simulink model "MATE_IEEE13Node"  (R2024b)
settings: Solver=FixedStepDiscrete  StartTime=0.0  StopTime=1  FixedStep=Ts  MaxStep=0.04  RelTol=1e-3
PostLoadFcn:
  | Ts=25e-6;
  | ieee_13NodesTestFeeder_init;
InitFcn:
  | Ts=25e-6;
  | ieee_13NodesTestFeeder_init;
undefined symbols (not defined in the file): C_603, C_604, C_605, C_607, ft2km, ieee_13NodesTestFeeder_init, L_603, L_604, L_605, L_607, R_603, R_604, R_605, R_607
libraries: simetranss x39, ee_lib x13, fl_lib x3, nesl_utility x3
Description:
  | Copyright 2008-2017 The MathWorks, Inc.
settings Model: ModifiedByFormat=Kyle Diller  Creator=Kyle Diller  LastModifiedBy=Kyle Diller
settings SolverCC: AlgebraicLoopSolver=TrustRegion
settings DataIOCC: ExternalInput=getinputstruct(op_IEEE_13_node_5)  InitialState=getstatestruct(op_IEEE_13_node_5)  LimitDataPoints=on  SaveFormat=Array  SignalLoggingSaveFormat=ModelDataLogs  ReturnWorkspaceOutputs=off
settings OptimizationCC: ExpressionDepthLimit=2147483647  LifeSpan=inf
settings DebuggingCC: AlgebraicLoopMsg=none  UnderspecifiedInitializationDetection=Classic  MergeDetectMultiDrivingBlocksExec=none  FcnCallInpInsideContextMsg=warning  AllowSymbolicDim=off  StateNameClashWarn=warning  SFUnexpectedBacktrackingDiag=warning  SFNoUnconditionalDefaultTransitionDiag=warning  SFExecutionAtInitializationDiag=none  ArithmeticOperatorsInVariantConditions=warning
settings HardwareCC: ProdBitPerPointer=32  ProdBitPerSizeT=32  ProdBitPerPtrDiffT=32  ProdLargestAtomicFloat=None  ProdIntDivRoundTo=Undefined  ProdEndianess=Unspecified  ProdWordSize=32  ProdHWDeviceType=32-bit Generic
settings ModelReferenceCC: EnableRefExpFcnMdlSchedulingChecks=on  PropagateSignalLabelsOutOfModel=off
settings SFSimCC: SimUseLocalCustomCode=off  CustomCodeUndefinedFunction=UseInterfaceOnly
settings RTWCC: RTWUseLocalCustomCode=off  GPUComputeCapability=3.5
settings CodeAppCC: StateflowObjectComments=on
settings GRTTargetCC: TargetLangStandard=C89/C90 (ANSI)  CombineOutputUpdateFcns=off  GRTInterface=on
settings ConfigComp: CovMetricSettings=dw  CovSaveCumulativeToWorkspaceVar=on  CovSaveSingleToWorkspaceVar=on  CovExternalEMLEnable=off  CovSFcnEnable=off
settings SimscapeCC: SimscapeNormalizeSystem=off

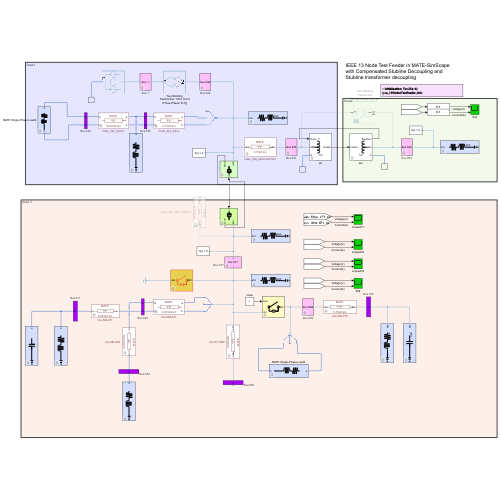
[thumbnail: Simulink's stored preview of the top-level diagram]
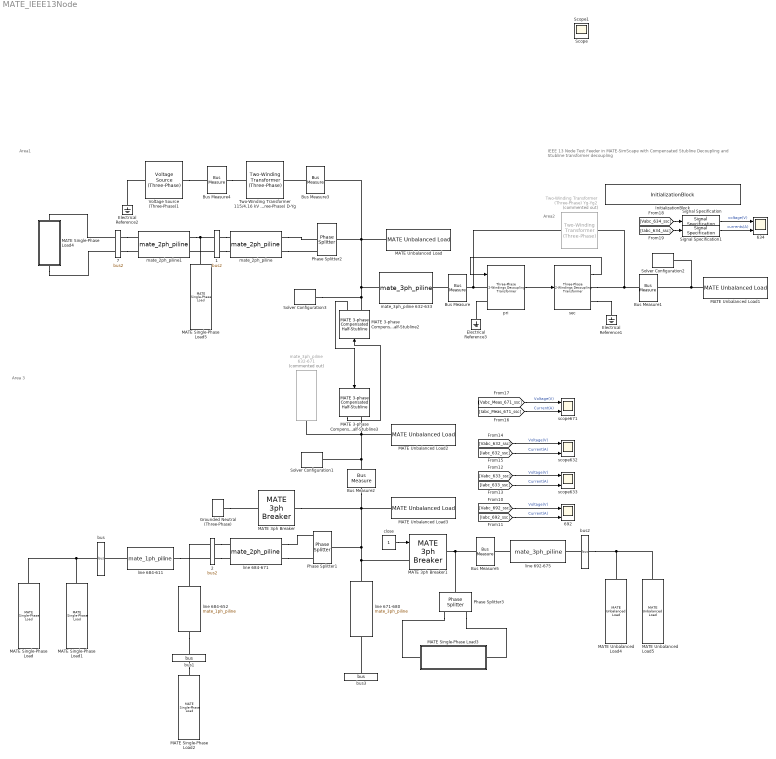
== system MATE_IEEE13Node ==
  note: IEEE 13 Node Test Feeder in MATE-SimScape
      | with Compensated Stubline Decoupling and
      | Stubline transformer decoupling
  note: Area1
  note: Area2
  note: Area 3
  1 : simetranss/Measure/bus2  bn=645
      settings: AttributesFormatString=Bus %<bn>
  2 : simetranss/Measure/bus2  bn=684
      settings: AttributesFormatString=Bus %<bn>
  634 : Scope  NumInputPorts=2
  692 : Scope  NumInputPorts=2
  7 : simetranss/Measure/bus2  bn=646
      settings: AttributesFormatString=Bus %<bn>
  Bus Measure : simetranss/Measure/Bus Measure  VoltageMeasurement=phase-to-phase  SetLabelV=on  LabelV=Vabc_633_ssc  Vpu=off  VpuLL=off  CurrentMeasurement=yes  SetLabelI=on  LabelI=Iabc_633_ssc  Ipu=off  Pbase=100e6  Vbase=500e3  bnumber=633  dis=off
      settings: AttributesFormatString=Bus %<bnumber>
  Bus Measure1 : simetranss/Measure/Bus Measure  VoltageMeasurement=phase-to-phase  SetLabelV=on  LabelV=Vabc_634_ssc  Vpu=off  VpuLL=off  CurrentMeasurement=yes  SetLabelI=on  LabelI=Iabc_634_ssc  Ipu=off  Pbase=100e6  Vbase=500e3  bnumber=634  dis=off
      settings: AttributesFormatString=Bus %<bnumber>
  Bus Measure2 : simetranss/Measure/Bus Measure  VoltageMeasurement=phase-to-ground  SetLabelV=on  LabelV=Vabc_Meas_671_ssc  Vpu=off  VpuLL=off  CurrentMeasurement=yes  SetLabelI=on  LabelI=Iabc_Meas_671_ssc  Ipu=off  Pbase=100e6  Vbase=500e3  bnumber=671  dis=off
      settings: AttributesFormatString=Bus %<bnumber>
  Bus Measure3 : simetranss/Measure/Bus Measure  VoltageMeasurement=phase-to-ground  SetLabelV=on  LabelV=Vabc_632_ssc  Vpu=off  VpuLL=off  CurrentMeasurement=yes  SetLabelI=on  LabelI=Iabc_632_ssc  Ipu=off  Pbase=100e6  Vbase=500e3  bnumber=632  dis=off
      settings: AttributesFormatString=Bus %<bnumber>
  Bus Measure4 : simetranss/Measure/Bus Measure  VoltageMeasurement=phase-to-ground  SetLabelV=on  LabelV=V1  Vpu=off  VpuLL=off  CurrentMeasurement=yes  SetLabelI=on  LabelI=I1  Ipu=off  Pbase=100e6  Vbase=500e3  bnumber=1  dis=off
      settings: AttributesFormatString=Bus %<bnumber>
  Bus Measure5 : simetranss/Measure/Bus Measure  VoltageMeasurement=phase-to-ground  SetLabelV=on  LabelV=Vabc_692_ssc  Vpu=off  VpuLL=off  CurrentMeasurement=yes  SetLabelI=on  LabelI=Iabc_692_ssc  Ipu=off  Pbase=100e6  Vbase=500e3  bnumber=692  dis=off
      settings: AttributesFormatString=Bus %<bnumber>
  Electrical Reference1 : fl_lib/Electrical/Electrical Elements/Electrical Reference
  Electrical Reference2 : fl_lib/Electrical/Electrical Elements/Electrical Reference
  Electrical Reference3 : fl_lib/Electrical/Electrical Elements/Electrical Reference
  Grounded Neutral (Three-Phase) : ee_lib/Connectors & References/Grounded Neutral (Three-Phase)
  InitializationBlock : simetranss/Usefulls/InitializationBlock  InitVar=Ts=25e-6;  InitFile=ieee_13NodesTestFeeder_init;  prel=off  posl=on  inif=on
  MATE 3-phase Compensated Half-Stubline2 : simetranss/Network decoupling/MATE 3-phase Compensated Half-Stubline  stype=3-phase coupled line (1 mode)  FF=60  RR=R_601  LL=L_601  CC=C_601  len=2000*ft2km  Ts=Ts  comp=on  stdel=off
  MATE 3-phase Compensated Half-Stubline3 : simetranss/Network decoupling/MATE 3-phase Compensated Half-Stubline  stype=3-phase coupled line (1 mode)  FF=60  RR=R_601  LL=L_601  CC=C_601  len=2000*ft2km  Ts=Ts  comp=off  stdel=off
  MATE 3ph Breaker : simetranss/Switches/MATE 3ph Breaker  InitialState=open  SwitchA=on  SwitchB=off  SwitchC=off  SwitchTimes=[0.2 0.25]  External=off  BreakerResistance=0.01  Roff=1e9  SnubberResistance=1e6  SnubberCapacitance=inf
  MATE 3ph Breaker1 : simetranss/Switches/MATE 3ph Breaker  InitialState=open  SwitchA=on  SwitchB=off  SwitchC=off  SwitchTimes=[0.2 0.25]  External=on  BreakerResistance=0.01  Roff=0  SnubberResistance=1e6  SnubberCapacitance=inf
  MATE Single-Phase Load : simetranss/Passive/MATE Single-Phase Load  Vabc=4160/sqrt(3)  Fn=60  typ=Capacitance  Pabc=[160 ]*1e3  QLabc=[ 90]*1e3  QCabc=100e3
  MATE Single-Phase Load1 : simetranss/Passive/MATE Single-Phase Load  Vabc=4160/sqrt(3)  Fn=60  typ=Series RL  Pabc=170e3  QLabc=80e3  QCabc=100e3
  MATE Single-Phase Load2 : simetranss/Passive/MATE Single-Phase Load  Vabc=4160/sqrt(3)  Fn=60  typ=Series RL  Pabc=128e3  QLabc=86e3  QCabc=100e3
  MATE Single-Phase Load3 : Subsystem  AncestorBlock=simetranss/Passive/MATE Single-Phase Load  mask(MATE 1-phase load){Vabc=1.71484*2401.78, Fn=60, typ=Series RL, Pabc=170e3, QLabc=151e3, QCabc=100e3}
      mask prompts: Vabc "Nominal voltage (Vrms)"; Fn "Nominal frequency fn (Hz):"; typ "Load type"; Pabc "Active powers (W)"; QLabc "Inductive reactive powers (positive var):"; QCabc "Capacitive reactive powers (positive var):"
      mask help: This block implements either a series RL load or a purely capacitive load.
      mask init:
      | block=gcb;
      | type=get_param(block,'typ');
      | 
      | if isequal (type,'Series RL')
      | j=sqrt(-1);
      | S=Pabc-j*QLabc;
      | Z=Vabc.*Vabc./S;
      | R=real(Z);
      | L=imag(Z)/2/pi/Fn;
      | 
      | s1 = 0;
      | s2 =-50;
      | s3 = 450;
      | s4 =50;
      | r1 = [0    30    30    38    53    68    83    98   113   120   120   150];
      | r2 =[0     0     0    25   -25    25   -25    25   -25     0     0     0];
      | c1 =[0];
      | c2 =[0 ];
      | c3 =[0];
      | c4 = [0];
      | c5=0;
      | c6=0;
      | l1 =[150   173   173   174   178   184   190   197   202   205   206   204   201 201   197   196   198   201   207   214   220   225   229   229   227   224   224   220   219   221   225   230   237   243   249   252   253   251   247  247   244   243   244   248   254   260   267   272   275   276   276   300 450];
      | l2 =[0     0     1    11    19    24    25    23    17     8    -2   -12   -18 -18    -9     1    11    19    24    25    23    17     8    -2   -12   -18 -18    -9     1    11    19    24    25    23    17     8    -2   -12   -18  -18    -9     1    11    19    24    25    23    17     8     0     0     0 0];
      | sca=0.5;
      | neutral=0;
      | ground=0;
      | else
      |     j=sqrt(-1);
      | S=QCabc;
      | Z=Vabc.*Vabc./S;
      | w=2*pi*Fn;
      | % Z=1/(wC)
      | C=1/w./Z;
      | 
      | 
      | s1 = 0;
      | s2 =-50;
      | s3 = 450;
      | s4 =50;
      | r1 = [0    ];
      | r2 =[0   ];
      | c1 =[450   390   390   393   395   393   390   390   393   395]-200;
      | c2 =[0     0     8    16    25    16     8    -8   -16   -25];
      | c3 =[360   360   360   250]-200;
      | c4 = [25   -25     0     0];
      | c5 =[ 455 200];
      | c6 = [0 0];
      | l1 =[0];
      | l2 =[0 ];
      | sca=0.5;
      | neutral=0;
      | 
      | ground=1;
      | 
      | 
      | 
      | end
      mask TypeOptions typ: Series RL | Capacitance
      mask Callback typ:
      | block = gcb;
      | type=get_param(block,'typ');
      | 
      | visib=get_param(block,'MaskVisibilities');
      | if isequal(type,'Series RL')
      |     visib{4}='on';;visib{5}='on';visib{6}='off';
      | else
      |     visib{4}='off';visib{5}='off';visib{6}='on';
      | end
      | set_param(block,'MaskVisibilities',visib);
      | 
      | 
      | if isequal(type,'Series RL')
      |     set_param([block '/RLseries'], 'Commented', 'off');
      |     set_param([block '/C'], 'Commented', 'on');
      | else
      |     set_param([block '/RLseries'], 'Commented', 'on');
      |     set_param([block '/C'], 'Commented', 'off');
      | end
      mask Display:
      | plot(s1-160,s2,s3+80,s4,r1,r2,l1,l2,c1,c2,c3,c4,c5,c6)
      | 
      | plot( ground*[s3,s3], ground*[-s2/4,s2/4])
      | plot( ground*[s3+30,s3+30], ground*[-s2/6,s2/6])
      | plot( ground*[s3+60,s3+60], ground*[-s2/10,s2/10])
      | 
      | plot( neutral*[s3,s3+80], neutral*[0,0])
  MATE Single-Phase Load4 : Subsystem  AncestorBlock=simetranss/Passive/MATE Single-Phase Load  mask(MATE 1-phase load){Vabc=4160, Fn=60, typ=Series RL, Pabc=170e3, QLabc=151e3, QCabc=100e3}
      mask prompts: Vabc "Nominal voltage (Vrms)"; Fn "Nominal frequency fn (Hz):"; typ "Load type"; Pabc "Active powers (W)"; QLabc "Inductive reactive powers (positive var):"; QCabc "Capacitive reactive powers (positive var):"
      mask help: This block implements either a series RL load or a purely capacitive load.
      mask init: same as MATE_IEEE13Node/MATE Single-Phase Load3
      mask TypeOptions typ: Series RL | Capacitance
      mask Callback typ:
      | block = gcb;
      | type=get_param(block,'typ');
      | 
      | visib=get_param(block,'MaskVisibilities');
      | if isequal(type,'Series RL')
      |     visib{4}='on';;visib{5}='on';visib{6}='off';
      | else
      |     visib{4}='off';visib{5}='off';visib{6}='on';
      | end
      | set_param(block,'MaskVisibilities',visib);
      | 
      | 
      | if isequal(type,'Series RL')
      |     set_param([block '/RLseries'], 'Commented', 'off');
      |     set_param([block '/C'], 'Commented', 'on');
      | else
      |     set_param([block '/RLseries'], 'Commented', 'on');
      |     set_param([block '/C'], 'Commented', 'off');
      | end
      mask Display:
      | plot(s1-160,s2,s3+80,s4,r1,r2,l1,l2,c1,c2,c3,c4,c5,c6)
      | 
      | plot( ground*[s3,s3], ground*[-s2/4,s2/4])
      | plot( ground*[s3+30,s3+30], ground*[-s2/6,s2/6])
      | plot( ground*[s3+60,s3+60], ground*[-s2/10,s2/10])
      | 
      | plot( neutral*[s3,s3+80], neutral*[0,0])
  MATE Single-Phase Load5 : simetranss/Passive/MATE Single-Phase Load  Vabc=1.03283*4160/sqrt(3)  Fn=60  typ=Series RL  Pabc=170e3  QLabc=125e3  QCabc=100e3
  MATE Unbalanced Load : simetranss/Passive/MATE Unbalanced Load  Vabc=[ 1.021 1.042 1.0174]*2401.78  Fn=60  typ=Series RL  Pabc="[17 66  117]*1e3/2"  QLabc="[10 38  68]*1e3/2"  QCabc="[190  60  212]*1e3"
  MATE Unbalanced Load1 : simetranss/Passive/MATE Unbalanced Load  Vabc=[ 0.993926 1.02168 0.995885]*277.128  Fn=60  typ=Series RL  Pabc=[160 120 120]*1e3  QLabc=[110 90 90]*1e3  QCabc="[190  60  212]*1e3"
  MATE Unbalanced Load2 : simetranss/Passive/MATE Unbalanced Load  Vabc=[ 0.987076 1.0519 0.978043]*2401.78  Fn=60  typ=Series RL  Pabc="[17 66  117]*1e3/2"  QLabc="[10 38  68]*1e3/2"  QCabc="[190  60  212]*1e3"
  MATE Unbalanced Load3 : simetranss/Passive/MATE Unbalanced Load  Vabc=[ 1.73773 1.77224 1.71484]*2401.78  Fn=60  typ=Series RL  Pabc=[385 385 385 ]*1e3  QLabc=[220 220 220]*1e3  QCabc="[190  60  212]*1e3"
  MATE Unbalanced Load4 : simetranss/Passive/MATE Unbalanced Load  Vabc=[ 0.98063 1.05431 0.975983]*2401.78  Fn=60  typ=Series RL  Pabc="[485  68  290]*1e3"  QLabc="[190  60  212]*1e3"  QCabc="[190  60  212]*1e3"
  MATE Unbalanced Load5 : simetranss/Passive/MATE Unbalanced Load  Vabc=[ 0.98063 1.05431 0.975983]*2401.78  Fn=60  typ=Capacitance  Pabc="[485  68  290]*1e3"  QLabc="[190  60  212]*1e3"  QCabc="[190  60  212]*1e3"
  Phase Splitter1 : ee_lib/Connectors & References/Phase Splitter
  Phase Splitter2 : ee_lib/Connectors & References/Phase Splitter
  Phase Splitter3 : ee_lib/Connectors & References/Phase Splitter
  Signal Specification : SignalSpecification  Dimensions=3
  Signal Specification1 : SignalSpecification  Dimensions=3
  Solver Configuration1 : nesl_utility/Solver Configuration  PhysicalDomain=network_engine_domain  SubClassName=solver  LeftPortType=input  RightPortType=generic  Tones=[]  Harmonics=[]  SimulateNoise=off  Profile=off  UseLocalSampling=off  EnableSwitchedLinearOptims=on  FrequencyDomain=off  UseCCode=off  RelTol=0.001  AbsTol=1e-06  MinStep=1e-09  ToWorkspace=off  RevertToSquareIcSolve=off  NumHomotopyIterations=100  PhasorMode=off  PhasorModeNumHarmonics=1  ConsistencySolver=NEWTON_FTOL  IndexReductionMethod=DerivativeReplacement  DoDC=off  ResidualTolerance=1e-09  ConsistencyTolSource=GLOBAL  ConsistencyAbsTol=0.001  ConsistencyRelTol=0.001  ConsistencyTolFactor=0.001  UseLocalSolver=on  LocalSolverChoice=NE_PARTITIONING_ADVANCER  ResolveIndetEquations=on  FunctionEvalNumThread=1  LocalSolverSampleTime=Ts  DoFixedCost=on  MaxNonlinIter=1  MaxModeIter=2  ComputeImpulses=off  ImpulseIterations=2  LinearAlgebra=auto  LinearAlgebraNumThread=0  EquationFormulation=NE_TIME_EF  DelaysMemoryBudget=1024  AutomaticFiltering=off  FilteringTimeConstant=0.001  PartitionStorageMethod=AS_NEEDED  PartitionMemoryBudget=1024  PartitionMethod=ROBUST  MultibodyUseLocalSolver=off  MultibodyLocalSolverChoice=ODE1  MultibodyLocalSolverSampleTime=0.001
  Solver Configuration2 : nesl_utility/Solver Configuration  PhysicalDomain=network_engine_domain  SubClassName=solver  LeftPortType=input  RightPortType=generic  Tones=[]  Harmonics=[]  SimulateNoise=off  Profile=off  UseLocalSampling=off  EnableSwitchedLinearOptims=on  FrequencyDomain=off  UseCCode=off  RelTol=0.001  AbsTol=1e-06  MinStep=1e-09  ToWorkspace=off  RevertToSquareIcSolve=off  NumHomotopyIterations=100  PhasorMode=off  PhasorModeNumHarmonics=1  ConsistencySolver=NEWTON_FTOL  IndexReductionMethod=DerivativeReplacement  DoDC=off  ResidualTolerance=1e-09  ConsistencyTolSource=GLOBAL  ConsistencyAbsTol=0.001  ConsistencyRelTol=0.001  ConsistencyTolFactor=0.001  UseLocalSolver=on  LocalSolverChoice=NE_PARTITIONING_ADVANCER  ResolveIndetEquations=on  FunctionEvalNumThread=1  LocalSolverSampleTime=Ts  DoFixedCost=on  MaxNonlinIter=1  MaxModeIter=2  ComputeImpulses=off  ImpulseIterations=2  LinearAlgebra=auto  LinearAlgebraNumThread=0  EquationFormulation=NE_TIME_EF  DelaysMemoryBudget=1024  AutomaticFiltering=off  FilteringTimeConstant=0.001  PartitionStorageMethod=AS_NEEDED  PartitionMemoryBudget=1024  PartitionMethod=ROBUST  MultibodyUseLocalSolver=off  MultibodyLocalSolverChoice=ODE1  MultibodyLocalSolverSampleTime=0.001
  Solver Configuration3 : nesl_utility/Solver Configuration  PhysicalDomain=network_engine_domain  SubClassName=solver  LeftPortType=input  RightPortType=generic  Tones=[]  Harmonics=[]  SimulateNoise=off  Profile=off  UseLocalSampling=off  EnableSwitchedLinearOptims=on  FrequencyDomain=off  UseCCode=off  RelTol=0.001  AbsTol=1e-06  MinStep=1e-09  ToWorkspace=off  RevertToSquareIcSolve=off  NumHomotopyIterations=100  PhasorMode=off  PhasorModeNumHarmonics=1  ConsistencySolver=NEWTON_FTOL  IndexReductionMethod=DerivativeReplacement  DoDC=off  ResidualTolerance=1e-09  ConsistencyTolSource=GLOBAL  ConsistencyAbsTol=0.001  ConsistencyRelTol=0.001  ConsistencyTolFactor=0.001  UseLocalSolver=on  LocalSolverChoice=NE_PARTITIONING_ADVANCER  ResolveIndetEquations=on  FunctionEvalNumThread=1  LocalSolverSampleTime=Ts  DoFixedCost=on  MaxNonlinIter=1  MaxModeIter=2  ComputeImpulses=off  ImpulseIterations=2  LinearAlgebra=auto  LinearAlgebraNumThread=0  EquationFormulation=NE_TIME_EF  DelaysMemoryBudget=1024  AutomaticFiltering=off  FilteringTimeConstant=0.001  PartitionStorageMethod=AS_NEEDED  PartitionMemoryBudget=1024  PartitionMethod=ROBUST  MultibodyUseLocalSolver=off  MultibodyLocalSolverChoice=ODE1  MultibodyLocalSolverSampleTime=0.001
  Two-Winding Transformer (Three-Phase) Yg-Yg2 : ee_lib/Passive/Transformers/Two-Winding Transformer (Three-Phase)  Commented=on  SRated=500e3 A*V  FRated=60 Hz  Winding1Connection=ee.enum.windingconnection.Yg  VRated1=4160 V  Winding2Connection=ee.enum.windingconnection.Yg  VRated2=480 V  CoreType=ee.enum.coretype.fivelimb  pu_Rw1=0.01  pu_Rw2=0.001  leakage_reactance_option=ee.enum.transformer_leakage.include  pu_Xl1=0.01  pu_Xl2=0.01  magnetizing_resistance_option=ee.enum.transformer_magnetizingResistance.exclude  pu_Rm=500  magnetizing_reactance_option=ee.enum.transformer_magnetizingReactance.exclude  saturation_option=ee.enum.transformer_saturation.exclude  pu_Xm=500  current_data=[0, .002, 1, 2]  magnetic_flux_data=[0, 1.2, 1.5, 1.51]  pu_X0=5000  i1_specify=off  i1_priority=None  i1=[0, 0, 0] A  i1_nominal_specify=off  i1_nominal_value=1  i1_nominal_unit=A  i2_specify=off  i2_priority=None  i2=[0, 0, 0] A  i2_nominal_specify=off  i2_nominal_value=1  i2_nominal_unit=A  phi_specify=off  phi_priority=None  phi=[0, 0, 0]  phi_nominal_specify=off  phi_nominal_value=1  phi_nominal_unit=1  power_dissipated_specify=off  power_dissipated_priority=None  power_dissipated=0 W  power_dissipated_nominal_specify=off  power_dissipated_nominal_value=1  power_dissipated_nominal_unit=W
      settings: InternalSimscapePortConfiguration="{\"Bottom\":[],\"Left\":[{\"id\":\"N1\",\"label\":\"~1\",\"type\":\"foundation.electrical.three_phase\"}],\"Right\":[{\"id\":\"N2\",\"label\":\"~2\",\"type\":\"foundation.electrical.three_phase\"}],\"Top\":[]}"
  Two-Winding Transformer 115/4.16 kV (Three-Phase) D-Yg : ee_lib/Passive/Transformers/Two-Winding Transformer (Three-Phase)  SRated=5000e3 A*V  FRated=60 Hz  Winding1Connection=ee.enum.windingconnection.delta1  VRated1=115e3 V  Winding2Connection=ee.enum.windingconnection.Yg  VRated2=4160 V  CoreType=ee.enum.coretype.threelimb  pu_Rw1=0.00001  pu_Rw2=0.01  leakage_reactance_option=ee.enum.transformer_leakage.include  pu_Xl1=0.01  pu_Xl2=0.07  magnetizing_resistance_option=ee.enum.transformer_magnetizingResistance.include  pu_Rm=500  magnetizing_reactance_option=ee.enum.transformer_magnetizingReactance.include  saturation_option=ee.enum.transformer_saturation.exclude  pu_Xm=500  current_data=[0, .002, 1, 2]  magnetic_flux_data=[0, 1.2, 1.5, 1.51]  pu_X0=5000  i1_specify=off  i1_priority=None  i1=[0, 0, 0] A  i1_nominal_specify=off  i1_nominal_value=1  i1_nominal_unit=A  i2_specify=off  i2_priority=None  i2=[0, 0, 0] A  i2_nominal_specify=off  i2_nominal_value=1  i2_nominal_unit=A  phi_specify=off  phi_priority=None  phi=[0, 0, 0]  phi_nominal_specify=off  phi_nominal_value=1  phi_nominal_unit=1  power_dissipated_specify=off  power_dissipated_priority=None  power_dissipated=0 W  power_dissipated_nominal_specify=off  power_dissipated_nominal_value=1  power_dissipated_nominal_unit=W
      settings: InternalSimscapePortConfiguration="{\"Bottom\":[],\"Left\":[{\"id\":\"N1\",\"label\":\"~1\",\"type\":\"foundation.electrical.three_phase\"}],\"Right\":[{\"id\":\"N2\",\"label\":\"~2\",\"type\":\"foundation.electrical.three_phase\"}],\"Top\":[]}"
  Voltage Source (Three-Phase)1 : ee_lib/Sources/Voltage Source (Three-Phase)  vline_rms=115e3 V  shift=0 deg  freq=60 Hz  impedance_option=2  SShortCircuit=1e6 A*V  XR=15  R=0.0001 Ohm  L=3.97e-4 H  harmonic_option=0  harmonic_orders=[5, 7, 11, 13]  harmonic_ratios=[.1, .1, .1, .1]  G_parasitic=0 1/Ohm  I_specify=off  I_priority=None  I=[0, 0, 0] A  I_nominal_specify=off  I_nominal_value=1  I_nominal_unit=A
  bus : simetranss/Measure/bus  bn=611
      settings: AttributesFormatString=Bus %<bn>
  bus1 : simetranss/Measure/bus  bn=652
      settings: AttributesFormatString=Bus %<bn>
  bus2 : simetranss/Measure/bus  bn=675
      settings: AttributesFormatString=Bus %<bn>
  bus3 : simetranss/Measure/bus  bn=680
      settings: AttributesFormatString=Bus %<bn>
  close : Constant
  line 671-680 : simetranss/Lines/mate_3ph_piline  FF=60  conf=config 6  lenfeet=2500  dmi=on  RR33=R_601  LL33=L_601  CC33=C_601  lenkm=1000*ft2km
  line 684-611 : simetranss/Lines/mate_1ph_piline  FF=60  conf=config 9  lenfeet=1500  dmi=on  RR1=R_605(3,3)  LL1=L_605(3,3)  CC1=C_605(3,3)  lenkm=300*ft2km
  line 684-652 : simetranss/Lines/mate_1ph_piline  FF=60  conf=config 9  lenfeet=1500  dmi=on  RR1=R_607(1,1)  LL1=L_607(1,1)  CC1=C_607(1,1)  lenkm=800*ft2km
  line 684-671 : simetranss/Lines/mate_2ph_piline  FF=60  conf=config 7  lenfeet=300  dmi=on  RR22=R_604([1 3],[1 3])  LL22=L_604([1 3],[1 3])  CC22=C_604([1 3],[1 3])  lenkm=300*ft2km
  line 692-675 : simetranss/Lines/mate_3ph_piline  FF=60  conf=config 6  lenfeet=2500  dmi=on  RR33=R_606  LL33=L_606  CC33=C_606  lenkm=500*ft2km
  mate_2ph_piline : simetranss/Lines/mate_2ph_piline  FF=60  conf=config 7  lenfeet=300  dmi=on  RR22=R_603(2:3,2:3)  LL22=L_603(2:3,2:3)  CC22=C_603(2:3,2:3)  lenkm=500*ft2km
  mate_2ph_piline1 : simetranss/Lines/mate_2ph_piline  FF=60  conf=config 7  lenfeet=300  dmi=on  RR22=R_603(2:3,2:3)  LL22=L_603(2:3,2:3)  CC22=C_603(2:3,2:3)  lenkm=300*ft2km
  mate_3ph_piline 632-633 : simetranss/Lines/mate_3ph_piline  FF=60  conf=config 6  lenfeet=2500  dmi=on  RR33=R_602  LL33=L_602  CC33=C_602  lenkm=500*ft2km
  mate_3ph_piline 632-671 : simetranss/Lines/mate_3ph_piline  Commented=on  FF=60  conf=config 6  lenfeet=2500  dmi=on  RR33=R_601  LL33=L_601  CC33=C_601  lenkm=2000*ft2km
  pri : simetranss/Network decoupling/Three-Phase 2-Windings Decoupling Transformer  deconf=Primary side  stdel=off  Winding1Connection=Yg  Winding2Connection=Yg  Ts=Ts  UNITS=pu  NominalPower=[ 500e3 , 60 ]  Winding1=[ 4160 , 0.001 , 0.01 ]  Winding2=[ 480, 0.01 , 0.01 ]  Rm=500  Lm=500
  scope632 : Scope  NumInputPorts=2
  scope633 : Scope  NumInputPorts=2
  scope671 : Scope  NumInputPorts=2
  sec : simetranss/Network decoupling/Three-Phase 2-Windings Decoupling Transformer  deconf=Secondary side  stdel=off  Winding1Connection=Yg  Winding2Connection=Yg  Ts=Ts  UNITS=pu  NominalPower=[ 500e3 , 60 ]  Winding1=[ 4160 , 0.001 , 0.01 ]  Winding2=[ 480, 0.01 , 0.01 ]  Rm=500  Lm=500
  Scope : Scope
  Scope1 : Scope
  wires:
  close/1 -> MATE 3ph Breaker1/1
  [Vabc_632_ssc] -> scope632/1  "Voltage(V)"
  [Iabc_692_ssc] -> 692/2  "Current(A)"
  [Iabc_633_ssc] -> scope633/2  "Current(A)"
  [Vabc_633_ssc] -> scope633/1  "Voltage(V)"
  [Vabc_692_ssc] -> 692/1  "Voltage(V)"
  [Iabc_632_ssc] -> scope632/2  "Current(A)"
  MATE 3-phase Compensated Half-Stubline3/1 -> MATE 3-phase Compensated Half-Stubline2/1
  MATE 3-phase Compensated Half-Stubline2/1 -> MATE 3-phase Compensated Half-Stubline3/1
  [Vabc_Meas_671_ssc] -> scope671/1  "Voltage(V)"
  [Iabc_Meas_671_ssc] -> scope671/2  "Current(A)"
  [Vabc_634_ssc] -> Signal Specification/1
  [Iabc_634_ssc] -> Signal Specification1/1
  Signal Specification/1 -> 634/1  "voltage(V)"
  Signal Specification1/1 -> 634/2  "currents(A)"
  pri/1 -> sec/1
  sec/1 -> pri/1
  connections:
  Solver Configuration1/RConn1 -- MATE 3-phase Compensated Half-Stubline3/RConn1 -- mate_3ph_piline 632-671/RConn1 -- MATE Unbalanced Load2/LConn1 -- Bus Measure2/LConn1
  MATE 3ph Breaker/RConn1 -- Bus Measure2/RConn1 -- MATE Unbalanced Load3/LConn1 -- line 671-680/LConn1 -- MATE 3ph Breaker1/LConn1 -- Phase Splitter1/LConn1
  bus3/RConn1 -- line 671-680/RConn1
  line 684-671/RConn1 -- Phase Splitter1/RConn1
  line 684-671/RConn2 -- Phase Splitter1/RConn3
  2/RConn2 -- line 684-671/LConn2
  2/RConn1 -- line 684-671/LConn1
  line 684-611/RConn1 -- 2/LConn2
  line 684-611/LConn1 -- bus/LConn1
  line 684-652/LConn1 -- 2/LConn1
  line 684-652/RConn1 -- bus1/RConn1
  bus/RConn1 -- MATE Single-Phase Load1/LConn1 -- MATE Single-Phase Load/LConn1
  bus1/LConn1 -- MATE Single-Phase Load2/LConn1
  MATE 3ph Breaker1/RConn1 -- Bus Measure5/RConn1 -- Phase Splitter3/LConn1
  bus2/RConn1 -- line 692-675/RConn1
  bus2/LConn1 -- MATE Unbalanced Load5/LConn1 -- MATE Unbalanced Load4/LConn1
  mate_2ph_piline/RConn2 -- Phase Splitter2/RConn3
  1/RConn2 -- mate_2ph_piline/LConn2
  1/LConn2 -- mate_2ph_piline1/RConn2
  mate_2ph_piline1/RConn1 -- 1/LConn1 -- MATE Single-Phase Load5/LConn1
  7/RConn2 -- mate_2ph_piline1/LConn2
  7/RConn1 -- mate_2ph_piline1/LConn1
  MATE Single-Phase Load4/LConn1 -- 7/LConn1
  MATE Single-Phase Load4/RConn1 -- 7/LConn2
  sec/RConn1 -- Two-Winding Transformer (Three-Phase) Yg-Yg2/RConn1 -- Bus Measure1/LConn1
  MATE Unbalanced Load1/LConn1 -- Bus Measure1/RConn1 -- Solver Configuration2/RConn1
  Electrical Reference2/LConn1 -- Voltage Source (Three-Phase)1/LConn1
  Voltage Source (Three-Phase)1/RConn1 -- Bus Measure4/LConn1
  mate_2ph_piline/RConn1 -- Phase Splitter2/RConn2
  1/RConn1 -- mate_2ph_piline/LConn1
  Bus Measure/LConn1 -- mate_3ph_piline 632-633/RConn1
  Grounded Neutral (Three-Phase)/LConn1 -- MATE 3ph Breaker/LConn1
  Phase Splitter3/RConn3 -- MATE Single-Phase Load3/LConn1
  Phase Splitter3/RConn1 -- MATE Single-Phase Load3/RConn1
  Bus Measure4/RConn1 -- Two-Winding Transformer 115/4.16 kV (Three-Phase) D-Yg/LConn1
  line 692-675/LConn1 -- Bus Measure5/LConn1
  MATE Unbalanced Load/LConn1 -- Solver Configuration3/RConn1 -- MATE 3-phase Compensated Half-Stubline2/RConn1 -- mate_3ph_piline 632-633/LConn1 -- Bus Measure3/LConn1 -- Phase Splitter2/LConn1
  Bus Measure3/RConn1 -- Two-Winding Transformer 115/4.16 kV (Three-Phase) D-Yg/RConn1
  sec/RConn2 -- Electrical Reference1/LConn1
  pri/LConn1 -- Two-Winding Transformer (Three-Phase) Yg-Yg2/LConn1 -- Bus Measure/RConn1
  Electrical Reference3/LConn1 -- pri/LConn2

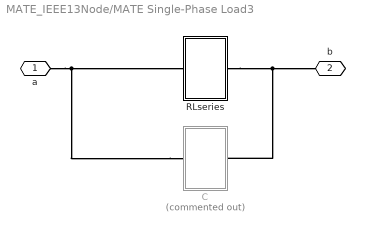
== system MATE_IEEE13Node/MATE Single-Phase Load3 ==
  C : Subsystem  Commented=on
  RLseries : Subsystem
  a : PMIOPort  Side=Left
  b : PMIOPort  Port=2  Side=Right
  connections:
  C/LConn1 -- a/RConn1 -- RLseries/LConn1
  RLseries/RConn1 -- C/RConn1 -- b/RConn1

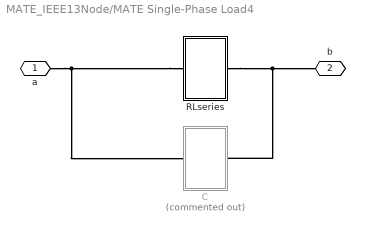
== system MATE_IEEE13Node/MATE Single-Phase Load4 ==
  C : Subsystem  Commented=on
  RLseries : Subsystem
  a : PMIOPort  Side=Left
  b : PMIOPort  Port=2  Side=Right
  connections:
  C/RConn1 -- RLseries/RConn1 -- b/RConn1
  RLseries/LConn1 -- a/RConn1 -- C/LConn1

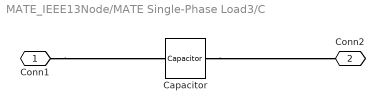
== system MATE_IEEE13Node/MATE Single-Phase Load3/C ==
  Capacitor : ee_lib/Passive/Capacitor  cap_option=ee.enum.passive.capacitor.capOption.const  c=C(1) F  Cvec=[1e-05, 1e-06] F  Vvec=[0, 10] V  CV_table_symmetry=ee.enum.passive.capacitor.tableSymmetry.yes  f_vec=[1, 10] kHz  DFext_vec=[.8, 1.2]  enable_C_tol=ee.enum.toleranceApplication.none  averaging_period=0 s  C_tol=5  tol_distribution=ee.enum.toleranceDistribution.uniform  nSigma=4  r=0 Ohm  g=0 1/Ohm  enable_operating_limits=ee.enum.enable.no  operating_limit_action=ee.enum.passive.reportOpLim.warn  max_working_voltage_range=[-25, 25] V  power_rating=1 W  maxTemperature=85 degC  thermalEnable=false  thermalMass=1 J/K  fault_action=simscape.enum.assert.action.none  t_fault=1 s  i_specify=off  i_priority=None  i=0 A  i_nominal_specify=off  i_nominal_value=1  i_nominal_unit=A  v_specify=off  v_priority=None  v=0 V  v_nominal_specify=off  v_nominal_value=1  v_nominal_unit=V  vc_specify=off  vc_priority=High  vc=0 V  vc_nominal_specify=off  vc_nominal_value=1  vc_nominal_unit=V  T_specify=off  T_priority=None  T=298.15 K  T_nominal_specify=off  T_nominal_value=1  T_nominal_unit=K
  Conn1 : PMIOPort  Side=Left
  Conn2 : PMIOPort  Port=2  Side=Right
  connections:
  Conn1/RConn1 -- Capacitor/LConn1
  Capacitor/RConn1 -- Conn2/RConn1

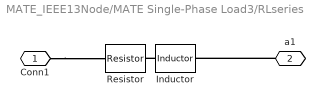
== system MATE_IEEE13Node/MATE Single-Phase Load3/RLseries ==
  Inductor : ee_lib/Passive/Inductor  l=L(1) H  enable_L_tol=ee.enum.toleranceApplication.none  L_tol=20  tol_distribution=ee.enum.toleranceDistribution.uniform  nSigma=4  r=0 Ohm  g=1e-9 1/Ohm  enable_operating_limits=ee.enum.enable.no  operating_limit_action=ee.enum.passive.reportOpLim.warn  max_working_current=1 A  power_rating=1 W  fault_action=simscape.enum.assert.action.none  t_fault=1 s  i_L_specify=off  i_L_priority=High  i_L=0 A  i_L_nominal_specify=off  i_L_nominal_value=1  i_L_nominal_unit=A
  Resistor : ee_lib/Passive/Resistor  R=R(1) Ohm  enable_R_tol=ee.enum.toleranceApplication.none  R_tol=5  tol_distribution=ee.enum.toleranceDistribution.uniform  nSigma=4  enable_operating_limits=ee.enum.enable.no  operating_limit_action=ee.enum.passive.reportOpLim.warn  power_rating=1 W  max_working_voltage=100 V  noise_mode=ee.enum.sources.noise.Disabled  Tdevice=25 degC  sample_time=1e-3 s  repeatability=ee.enum.ic.repeatability.notRepeatable  user_seed=0  auto_seed=717982854  fault_action=simscape.enum.assert.action.none  t_fault=1 s  power_derating_T1=70 degC  power_derating_T2=155 degC  operating_temperature_range_vec=[-50, 150] degC  alpha=3.93e-3 1/K  Tmeas=25 degC  thermal_mass=100 J/K  temperature_specify=off  temperature_priority=High  temperature=298.15 K  temperature_nominal_specify=off  temperature_nominal_value=1  temperature_nominal_unit=K
  Conn1 : PMIOPort  Side=Left
  a1 : PMIOPort  Port=2  Side=Right
  connections:
  Inductor/LConn1 -- Resistor/RConn1
  a1/RConn1 -- Inductor/RConn1
  Conn1/RConn1 -- Resistor/LConn1

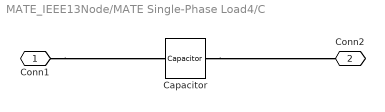
== system MATE_IEEE13Node/MATE Single-Phase Load4/C ==
  Capacitor : ee_lib/Passive/Capacitor  cap_option=ee.enum.passive.capacitor.capOption.const  c=C(1) F  Cvec=[1e-05, 1e-06] F  Vvec=[0, 10] V  CV_table_symmetry=ee.enum.passive.capacitor.tableSymmetry.yes  f_vec=[1, 10] kHz  DFext_vec=[.8, 1.2]  enable_C_tol=ee.enum.toleranceApplication.none  averaging_period=0 s  C_tol=5  tol_distribution=ee.enum.toleranceDistribution.uniform  nSigma=4  r=0 Ohm  g=0 1/Ohm  enable_operating_limits=ee.enum.enable.no  operating_limit_action=ee.enum.passive.reportOpLim.warn  max_working_voltage_range=[-25, 25] V  power_rating=1 W  maxTemperature=85 degC  thermalEnable=false  thermalMass=1 J/K  fault_action=simscape.enum.assert.action.none  t_fault=1 s  i_specify=off  i_priority=None  i=0 A  i_nominal_specify=off  i_nominal_value=1  i_nominal_unit=A  v_specify=off  v_priority=None  v=0 V  v_nominal_specify=off  v_nominal_value=1  v_nominal_unit=V  vc_specify=off  vc_priority=High  vc=0 V  vc_nominal_specify=off  vc_nominal_value=1  vc_nominal_unit=V  T_specify=off  T_priority=None  T=298.15 K  T_nominal_specify=off  T_nominal_value=1  T_nominal_unit=K
  Conn1 : PMIOPort  Side=Left
  Conn2 : PMIOPort  Port=2  Side=Right
  connections:
  Capacitor/RConn1 -- Conn2/RConn1
  Conn1/RConn1 -- Capacitor/LConn1

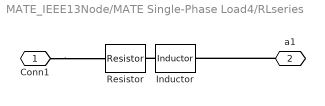
== system MATE_IEEE13Node/MATE Single-Phase Load4/RLseries ==
  Inductor : ee_lib/Passive/Inductor  l=L(1) H  enable_L_tol=ee.enum.toleranceApplication.none  L_tol=20  tol_distribution=ee.enum.toleranceDistribution.uniform  nSigma=4  r=0 Ohm  g=1e-9 1/Ohm  enable_operating_limits=ee.enum.enable.no  operating_limit_action=ee.enum.passive.reportOpLim.warn  max_working_current=1 A  power_rating=1 W  fault_action=simscape.enum.assert.action.none  t_fault=1 s  i_L_specify=off  i_L_priority=High  i_L=0 A  i_L_nominal_specify=off  i_L_nominal_value=1  i_L_nominal_unit=A
  Resistor : ee_lib/Passive/Resistor  R=R(1) Ohm  enable_R_tol=ee.enum.toleranceApplication.none  R_tol=5  tol_distribution=ee.enum.toleranceDistribution.uniform  nSigma=4  enable_operating_limits=ee.enum.enable.no  operating_limit_action=ee.enum.passive.reportOpLim.warn  power_rating=1 W  max_working_voltage=100 V  noise_mode=ee.enum.sources.noise.Disabled  Tdevice=25 degC  sample_time=1e-3 s  repeatability=ee.enum.ic.repeatability.notRepeatable  user_seed=0  auto_seed=456195728  fault_action=simscape.enum.assert.action.none  t_fault=1 s  power_derating_T1=70 degC  power_derating_T2=155 degC  operating_temperature_range_vec=[-50, 150] degC  alpha=3.93e-3 1/K  Tmeas=25 degC  thermal_mass=100 J/K  temperature_specify=off  temperature_priority=High  temperature=298.15 K  temperature_nominal_specify=off  temperature_nominal_value=1  temperature_nominal_unit=K
  Conn1 : PMIOPort  Side=Left
  a1 : PMIOPort  Port=2  Side=Right
  connections:
  Conn1/RConn1 -- Resistor/LConn1
  a1/RConn1 -- Inductor/RConn1
  Inductor/LConn1 -- Resistor/RConn1
